simulink model "lowPassFilter"  (R2024b)
settings: Solver=FixedStepAuto  StartTime=0.0  StopTime=Tend  FixedStep=0.0001  RelTol=1e-4
values from neighbouring files (symbols this model uses):
  omega_lpf = 2*pi*f_lpf    (= 628.318530718)    [setup.m]
  Ts = 1e-4    (= 0.0001)    [setup.m]    (also in test.m = 0.001)
settings Model: Creator=puroh  LastModifiedBy=tnoguchi
settings DataIOCC: SaveOutput=off  SaveTime=off
settings OptimizationCC: DefaultParameterBehavior=Inlined  EnhancedBackFolding=on  PassReuseOutputArgsAs=Individual arguments  ZeroExternalMemoryAtStartup=off  ZeroInternalMemoryAtStartup=off  OptimizeBlockOrder=speed  DifferentSizesBufferReuse=on  EfficientTunableParamExpr=on
settings DebuggingCC: ParameterTunabilityLossMsg=error  UnconnectedInputMsg=warning  UnconnectedOutputMsg=warning  UnconnectedLineMsg=warning
settings ModelReferenceCC: EnableRefExpFcnMdlSchedulingChecks=on
settings SFSimCC: MATLABDynamicMemAlloc=off
settings RTWCC: Description=Embedded Coder  SystemTargetFile=ert.tlc  TemplateMakefile=ert_default_tmf  GPUComputeCapability=3.5  DLArmComputeVersion=19.05
settings CodeAppCC: ForceParamTrailComments=on  IgnoreCustomStorageClasses=off  OperatorAnnotations=on  SimulinkDataObjDesc=on  SFDataObjDesc=on  InsertBlockDesc=on
settings ERTTargetCC: TargetLangStandard=C99 (ISO)  ERTCustomFileTemplate=example_file_process.tlc  DynamicArrayContainerType=coder::array
settings ConfigComp: CovBoundaryAbsTol=1.0e-5

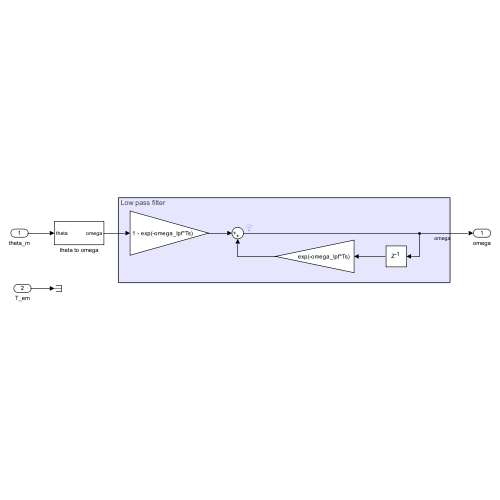
[thumbnail: Simulink's stored preview of the top-level diagram]
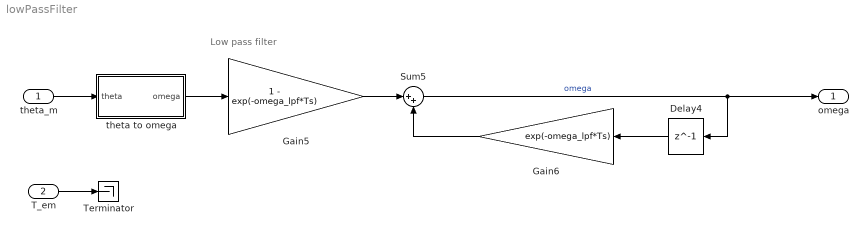
== system lowPassFilter ==
  note: Low pass filter
  theta_m : Inport  OutDataTypeStr=double  PortDimensions=1  SampleTime=[0.0001,0]
  T_em : Inport  Port=2  OutDataTypeStr=double  PortDimensions=1  SampleTime=[0.0001,0]
  Delay4 : Delay  DelayLength=1  InputProcessing=Columns as channels (frame based)
  Gain5 : Gain  Gain=1 - exp(-omega_lpf*Ts)
  Gain6 : Gain  Gain=exp(-omega_lpf*Ts)
  Sum5 : Sum  Inputs=|++
  Terminator : Terminator
  theta to omega : Subsystem
  omega : Outport  OutDataTypeStr=double  PortDimensions=1  SampleTime=[0.0001,0]
  wires:
  Delay4/1 -> Gain6/1
  Sum5/1 -> omega/1, Delay4/1  "omega"
  Gain5/1 -> Sum5/1
  Gain6/1 -> Sum5/2
  theta to omega/1(omega) -> Gain5/1
  theta_m/1 -> theta to omega/1(theta)
  T_em/1 -> Terminator/1

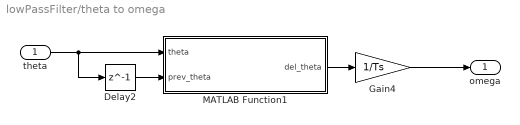
== system lowPassFilter/theta to omega ==
  theta : Inport
  Delay2 : Delay  DelayLength=1  InputProcessing=Columns as channels (frame based)
  Gain4 : Gain  Gain=1/Ts
  MATLAB Function1 : MATLAB Function  TreatAsAtomicUnit=on
  omega : Outport
  wires:
  Gain4/1 -> omega/1
  MATLAB Function1/1(del_theta) -> Gain4/1
  Delay2/1 -> MATLAB Function1/2(prev_theta)
  theta/1 -> Delay2/1, MATLAB Function1/1(theta)

== matlab function lowPassFilter/theta to omega/MATLAB Function1 ==
  data: theta input; del_theta output; prev_theta input
function del_theta = delta_theta(theta, prev_theta)

    % check if prev_theta exist before using to prevent error in 1st iteration 
    del_theta = theta - prev_theta;

    % prevent jumps in speed during 2pi to 0 transitions 
    while del_theta > pi
        del_theta = del_theta - 2*pi;
    end

    while del_theta < -pi
        del_theta = del_theta + 2*pi;
    end
    
end
